simulink subsystem "PvtSubSys_PLAN_ALC"  (R2020b)
settings: Solver=VariableStepAuto  StartTime=0.0  StopTime=10.0  RelTol=1e-3
undefined symbols (not defined in the file or in its folder): P_Global_WheelBase_m, P_Global_WheelTrack_m, P_PLAN_ALC_DPCConfirmTimeHMI, P_PLAN_ALC_DPCExtraMultiFrameConfirmCntDrv, P_PLAN_ALC_DPCExtraMultiFrameConfirmCntNoh, P_PLAN_ALC_DPCExtraMultiFrameConfirmCntOverTk, P_PLAN_ALC_DPCthresholdLcDrvLv1, P_PLAN_ALC_DPCthresholdLcDrvLv2, P_PLAN_ALC_DPCthresholdLcDrvLv3, P_PLAN_ALC_DynamicDPCthreshold, P_PLAN_ALC_FWheelPreTime, P_PLAN_ALC_LcCancelDPCThreshold, P_PLAN_ALC_LcCancelLaneChangeReqDspTimeCnt, P_PLAN_ALC_LcCancelRoadWidthOffset, P_PLAN_ALC_LcCancelRoadWidthOffsetForDPC, P_PLAN_ALC_LcCurvatureInhibitionValueBrkPoints, P_PLAN_ALC_LcCurvatureInhibitionValueTable, P_PLAN_ALC_LcDelayCntSetNoh, P_PLAN_ALC_LcDelayCntSetOverTk, P_PLAN_ALC_LCDeltaTmeGap, P_PLAN_ALC_LcDrv_DyDiffThreshold, P_PLAN_ALC_LcDrvHMILineValidFtime, P_PLAN_ALC_LcEnterLane_factor, P_PLAN_ALC_LcFinishDyDiffBrkPoint, P_PLAN_ALC_LcFinishDyDiffRwFactorForAP, P_PLAN_ALC_LcFinishDyDiffRwFactorForHMI, P_PLAN_ALC_LcFinishDyDiffTableValue, P_PLAN_ALC_LciDrvExistDefaultDisp, P_PLAN_ALC_LciOverTkDeltaSpdLv1, P_PLAN_ALC_LciOverTkDeltaSpdLv2, P_PLAN_ALC_LciOverTkDeltaSpdLv3, P_PLAN_ALC_LcOverTkDPCthreshold, P_PLAN_ALC_LcOverTkRearVehTTClimit, P_PLAN_ALC_NOHLcSwt, P_PLAN_ALC_NOHTurnSts, P_PLAN_ALC_OverTkCutOutDyRWFactor, P_PLAN_ALC_OveTkrSupDist, P_PLAN_ALC_PreCurvatureFactor, P_PLAN_ALC_PreCurvaturePreTime, P_PLAN_ALC_TurnLmpType, P_PLAN_ALC_vMinPreLC_Drv, P_PLAN_ALC_vMinPreLC_Noh, P_PLAN_ALC_vMinPreLC_OverTk, P_PLAN_LcCancelTestEnable, PLAN_ALC_DangerObjIndex, PLAN_ALC_LcCancelReason, PLAN_ALC_LcDecsLe, PLAN_ALC_LcDecsRi, PLAN_ALC_LcFeReason, PLAN_ALC_LcReason, PLAN_ALC_sts, PLAN_ALC_stsReason, PLAN_ALC_TurnLightReq
libraries: simulink x198, TrueDurationTime x21, RisingEdgeTimer x2, JumpDetectionUint x1
(part 2 of 4)

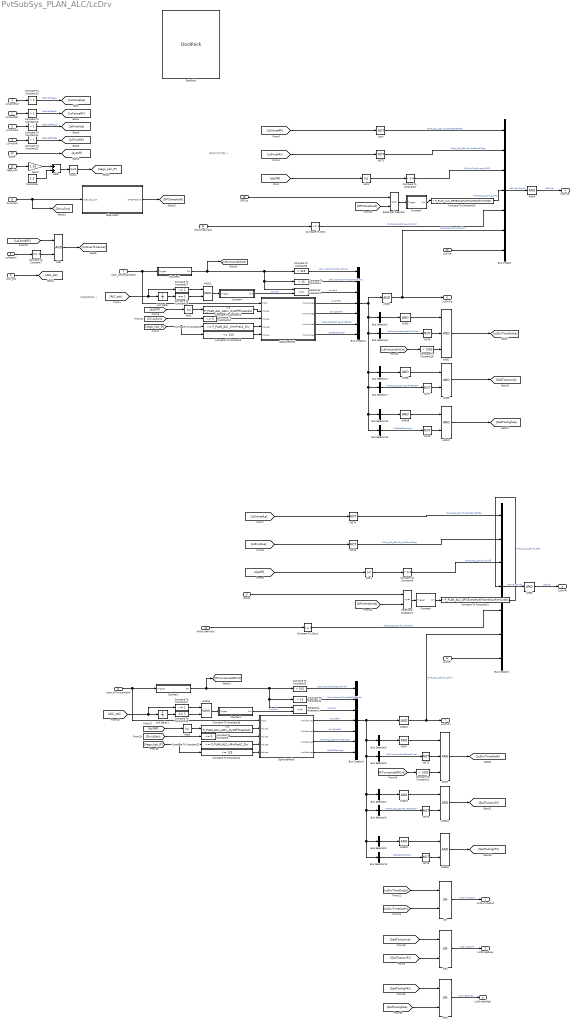
== system PvtSubSys_PLAN_ALC/LcDrv ==
  note: 换道可行性判断->
  note: 换道意图判断->
  LcCancelLe : Inport
  LcCancelRi : Inport  Port=2
  LcFinishLe : Inport  Port=3
  LcFinishRi : Inport  Port=4
  LcReason : Inport  Port=5
  ALC_sts : Inport  Port=6
  User_LeTurnLampON : Inport  Port=7
  User_RiTurnLampON : Inport  Port=8
  DrvLcSwt : Inport  Port=9
  dyDiff : Inport  Port=10
  HWALineLValid : Inport  Port=11
  HWALineRValid : Inport  Port=12
  LcAvLe : Inport  Port=13
  LcAvRi : Inport  Port=14
  Vego_kph : Inport  Port=15
  DPCLe : Inport  Port=16
  DPCRi : Inport  Port=17
  AND{,5,12,15,17} (5 alike) : Logic  AllPortsSameDT=off  OutDataTypeStr=boolean
  AND1 : Logic  Inputs=3  AllPortsSameDT=off  OutDataTypeStr=boolean
  AND{3,7..10,13,16,18} (8 alike) : Logic  Inputs=1  AllPortsSameDT=off  OutDataTypeStr=boolean
  AND11 : Logic  Operator=NAND  AllPortsSameDT=off  OutDataTypeStr=boolean
  AND14 : Logic  Operator=NAND  AllPortsSameDT=off  OutDataTypeStr=boolean
  AND2 : Logic  Inputs=3  AllPortsSameDT=off  OutDataTypeStr=boolean
  AND4 : Logic  Inputs=1  IconShape=distinctive  AllPortsSameDT=off  OutDataTypeStr=boolean
  AND6 : Logic  Inputs=1  IconShape=distinctive  AllPortsSameDT=off  OutDataTypeStr=boolean
  Abs{1..2,4..5} (4 alike) : Abs
  Add2 : Sum
  Bus Creator{,1..3} (4 alike) : BusCreator  Inputs=7
  Bus Selector1 : BusSelector  OutputSignals=LeTurnLampOnTimeNotTooShort,LciValid,DrvLcSwtON,PLAN_ALC_LcDrvLe_IPVehSpd,SpdNotTooHigh  OutputAsBus=on
  Bus Selector10 : BusSelector  OutputSignals=SpdNotTooHigh
  Bus Selector{2,4,9,11} (4 alike) : BusSelector  OutputSignals=LeTurnLampOnNotOverTime,LeTurnLampOnTimeNotTooShort,LciValid,DrvLcSwtON  OutputAsBus=on
  Bus Selector12 : BusSelector  OutputSignals=SpdNotTooHigh
  Bus Selector3 : BusSelector  OutputSignals=LeTurnLampOnTimeNotTooShort,LciValid,DrvLcSwtON,PLAN_ALC_LcDrvRi_IPVehSpd,SpdNotTooHigh  OutputAsBus=on
  Bus Selector5 : BusSelector  OutputSignals=PLAN_ALC_LcDrvRi_IPVehSpd
  Bus Selector6 : BusSelector  OutputSignals=LeTurnLampOnNotOverTime
  Bus Selector7 : BusSelector  OutputSignals=PLAN_ALC_LcDrvLe_IPVehSpd
  Bus Selector8 : BusSelector  OutputSignals=LeTurnLampOnNotOverTime
  Compare To Constant1 : simulink/Logic and Bit Operations/Compare To Constant  relop=<=  const=P_PLAN_ALC_LcDrv_DyDiffThreshold  OutDataTypeStr=boolean
  Compare To Constant10 : simulink/Logic and Bit Operations/Compare To Constant  relop=~=  const=0  OutDataTypeStr=boolean
  Compare To Constant11 : simulink/Logic and Bit Operations/Compare To Constant  relop=<  const=1000  OutDataTypeStr=boolean
  Compare To Constant12 : simulink/Logic and Bit Operations/Compare To Constant  relop=<=  const=125  OutDataTypeStr=boolean
  Compare To Constant{13..15,22} (4 alike) : simulink/Logic and Bit Operations/Compare To Constant  relop=>  const=1  OutDataTypeStr=boolean
  Compare To Constant16 : simulink/Logic and Bit Operations/Compare To Constant  relop=<  const=1000  OutDataTypeStr=boolean
  Compare To Constant17 : simulink/Logic and Bit Operations/Compare To Constant  relop=~=  const=1  OutDataTypeStr=boolean
  Compare To Constant18 : simulink/Logic and Bit Operations/Compare To Constant  relop=<=  const=P_PLAN_ALC_LcDrv_DyDiffThreshold  OutDataTypeStr=boolean
  Compare To Constant19 : simulink/Logic and Bit Operations/Compare To Constant  relop===  const=1  OutDataTypeStr=boolean
  Compare To Constant2 : simulink/Logic and Bit Operations/Compare To Constant  relop=>=  const=P_PLAN_ALC_vMinPreLC_Drv  OutDataTypeStr=boolean
  Compare To Constant20 : simulink/Logic and Bit Operations/Compare To Constant  relop=>  const=P_PLAN_ALC_DPCExtraMultiFrameConfirmCntDrv  OutDataTypeStr=boolean
  Compare To Constant21 : simulink/Logic and Bit Operations/Compare To Constant  relop=>  const=P_PLAN_ALC_DPCExtraMultiFrameConfirmCntDrv  OutDataTypeStr=boolean
  Compare To Constant23 : simulink/Logic and Bit Operations/Compare To Constant  relop=>=  const=P_PLAN_ALC_vMinPreLC_Drv  OutDataTypeStr=boolean
  Compare To Constant24 : simulink/Logic and Bit Operations/Compare To Constant  relop=>  const=15  OutDataTypeStr=boolean
  Compare To Constant25 : simulink/Logic and Bit Operations/Compare To Constant  relop=<  const=515  OutDataTypeStr=boolean
  Compare To Constant27 : simulink/Logic and Bit Operations/Compare To Constant  relop=~=  const=1  OutDataTypeStr=boolean
  Compare To Constant28 : simulink/Logic and Bit Operations/Compare To Constant  relop===  const=1  OutDataTypeStr=boolean
  Compare To Constant3 : simulink/Logic and Bit Operations/Compare To Constant  relop=<=  const=125  OutDataTypeStr=boolean
  Compare To Constant4 : simulink/Logic and Bit Operations/Compare To Constant  relop=>  const=15  OutDataTypeStr=boolean
  Compare To Constant5 : simulink/Logic and Bit Operations/Compare To Constant  relop=<  const=0.4  OutDataTypeStr=boolean
  Compare To Constant6 : simulink/Logic and Bit Operations/Compare To Constant  relop=<  const=0.4  OutDataTypeStr=boolean
  Compare To Constant7 : simulink/Logic and Bit Operations/Compare To Constant  relop===  const=4  OutDataTypeStr=boolean
  Compare To Constant8 : simulink/Logic and Bit Operations/Compare To Constant  relop=<  const=515  OutDataTypeStr=boolean
  Compare To Constant9 : simulink/Logic and Bit Operations/Compare To Constant  relop=~=  const=0  OutDataTypeStr=boolean
  Compare To Zero : simulink/Logic and Bit Operations/Compare To Zero  relop=~=  OutDataTypeStr=boolean
  Compare To Zero1 : simulink/Logic and Bit Operations/Compare To Zero  relop=~=  OutDataTypeStr=boolean
  Constant6 : Constant  Value=1.3  OutDataTypeStr=single
  Counter1 : Subsystem
  Counter2 : Subsystem
  Counter3 : Subsystem
  Counter4 : Subsystem
  Counter5 : Subsystem
  Counter6 : Subsystem
  DocBlock : simulink/Model-Wide Utilities/DocBlock  DocumentType=Text
      content=|
      | 模块说明：
      | 该模块用于计算是否触发拨杆换道，换道条件如下：
      |
      | 当如下条件全部满足左换道可行
      | 1.手动换道开关开启；
      | 2.车身中心距离车道中心线0.4m以内；
      | 3.仪表车速大于等于40kmh；
      | 4.左侧车道安全，换道过程中无碰撞风险；
      | 5.左侧车道控制线有效；
      | 6.3s内未发生右换道取消；
      | 7.3s内未发生右换道完成；
      | 8.左侧转向灯开关开启时（上升沿）开始计时，关闭左转向灯时或车辆中心距离控制线>0.8m或状态跳转到非Cruise（上升沿）时停止计时，计时满0.3s但不超过10s；
      |
      | 当如下条件全部满足则满足右换道可行
      | 1.手动换道开关开启；
      | 2.车身中心距离本车道中心线0.4m以内；
      | 3.仪表车速大于等于40kmh；
      | 4.左侧车道安全，换道过程中无碰撞风险；
      | 5.左侧车道控制线有效；
      | 6.3s内未发生左换道取消；
      | 7.3s内未发生左换道完成；
      | 8.右侧转向灯开关开启时（上升沿）开始计时，关闭右转向灯时或车辆中心距离控制线>0.8m或状态跳转到非Cruise（上升沿）时停止计时，计时满0.3s但不超过10s；
  Gain2 : Gain  Gain=1.03
  NOT{,1..9} (10 alike) : Logic  Operator=NOT  IconShape=distinctive  AllPortsSameDT=off  OutDataTypeStr=boolean
  OR : Logic  Operator=OR  AllPortsSameDT=off  OutDataTypeStr=boolean
  OR1 : Logic  Operator=OR  AllPortsSameDT=off  OutDataTypeStr=boolean
  OR2 : Logic  Operator=OR  AllPortsSameDT=off  OutDataTypeStr=boolean
  Relational Operator{,1..3} (4 alike) : RelationalOperator  Operator=<=  OutDataTypeStr=boolean  RndMeth=Simplest
  Round : Rounding  Operator=round
  SigValueHold1 : Stateflow chart  TreatAsAtomicUnit=on
  SigValueHold3 : Stateflow chart  TreatAsAtomicUnit=on
  Subsystem : Subsystem
  Unit Delay : UnitDelay  SampleTime=-1  HasFrameUpgradeWarning=on
  Unit Delay1 : UnitDelay  SampleTime=-1  HasFrameUpgradeWarning=on
  LciDrvTimeOut : Outport
  LciDrvSpdLow : Outport  Port=2
  LciDrvSpdHigh : Outport  Port=3
  LcDrvLe : Outport  Port=4
  LcDrvRi : Outport  Port=5
  LciDrvLe : Outport  Port=6
  LciDrvRi : Outport  Port=7
  wires:
  LcAvRi/1 -> Bus Creator1/7
  LcAvLe/1 -> Bus Creator/7
  OR2/1 -> LciDrvSpdHigh/1  "LciDrvSpdHigh"
  [SpdToohighLe] -> OR2/2
  [SpdToohighRi] -> OR2/1
  AND18/1 -> AND17/1
  NOT9/1 -> AND17/2
  Bus Selector11/1 -> AND18/1
  Bus Selector12/1 -> NOT9/1  "<SpdNotTooHigh>"
  AND17/1 -> [SpdToohighLe]
  Bus Creator2/1 -> AND3/1, Bus Selector1/1, Bus Selector8/1, Bus Selector2/1, Bus Selector7/1, Bus Selector11/1, Bus Selector12/1
  Bus Creator3/1 -> Bus Selector3/1, Bus Selector6/1, Bus Selector4/1, Bus Selector5/1, Bus Selector10/1, Bus Selector9/1, AND10/1
  AND15/1 -> [SpdToohighRi]
  Bus Selector10/1 -> NOT8/1  "<SpdNotTooHigh>"
  Bus Selector9/1 -> AND16/1
  NOT8/1 -> AND15/2
  AND16/1 -> AND15/1
  AND/1 -> [LcOverTkCancel]
  Compare To Constant7/1 -> AND/2
  [LcCancelRi] -> AND/1
  LcReason/1 -> Compare To Constant7/1
  Bus Creator1/1 -> AND6/1  "LcDrvRi_Conds"
  AND6/1 -> LcDrvRi/1  "LcDrvRi"
  AND4/1 -> LcDrvLe/1  "LcDrvLe"
  OR/1 -> LciDrvTimeOut/1  "LciDrvTimeOut"
  [LciDrvTimeOutRi] -> OR/2
  [LciDrvTimeOutLe] -> OR/1
  Bus Creator/1 -> AND4/1  "LcDrvLe_Conds"
  [LcFinishLe] -> NOT5/1
  [LcCancelLe] -> NOT4/1
  [LcFinishRi] -> NOT1/1
  NOT/1 -> Bus Creator/1  "PLAN_ALC_LcDrvLe_NoLcCancelFlag"
  LcFinishLe/1 -> Compare To Constant14/1
  LcFinishRi/1 -> Compare To Constant22/1
  LcCancelRi/1 -> Compare To Constant15/1
  Compare To Constant5/1 -> Bus Creator1/3  "PLAN_ALC_LcDrvRi_dyDiff"
  Abs4/1 -> Compare To Constant5/1
  [dyDiff] -> Abs4/1
  NOT5/1 -> Bus Creator1/2  "PLAN_ALC_LcDrvRi_NoLcFinishFlag"
  NOT4/1 -> Bus Creator1/1  "PLAN_ALC_LcDrvRi_NoLcCancelFlag"
  NOT1/1 -> Bus Creator/2  "PLAN_ALC_LcDrvLe_NoLcFinishFlag"
  [LcCancelRi] -> NOT/1
  [dyDiff] -> Abs1/1
  dyDiff/1 -> [dyDiff]
  LcCancelLe/1 -> Compare To Constant13/1
  HWALineRValid/1 -> Compare To Zero1/1
  Abs1/1 -> Compare To Constant6/1
  Compare To Constant6/1 -> Bus Creator/3  "PLAN_ALC_LcDrvLe_dyDiff"
  Compare To Constant20/1 -> Bus Creator/4  "PLAN_ALC_LcDrvLe_DPC"
  HWALineLValid/1 -> Compare To Zero/1
  [DPCthreshold] -> Relational Operator1/2
  Compare To Zero1/1 -> Bus Creator1/5  "PLAN_ALC_LcDrvRi_LineValid"
  Relational Operator1/1 -> Counter6/1(Trigger)
  DPCLe/1 -> Relational Operator/1
  DPCRi/1 -> Relational Operator1/1
  [DPCthreshold] -> Relational Operator/2
  Compare To Zero/1 -> Bus Creator/5  "PLAN_ALC_LcDrvLe_LineValid"
  [SpdTooLowLe] -> OR1/1
  [SpdTooLowRi] -> OR1/2
  OR1/1 -> LciDrvSpdLow/1  "LciDrvSpdLow"
  Compare To Constant13/1 -> [LcCancelLe]  "LcFinishFlagLe"
  Compare To Constant15/1 -> [LcCancelRi]  "LcFinishFlagRi"
  Compare To Constant14/1 -> [LcFinishLe]  "LcCancelFlagLe"
  Compare To Constant22/1 -> [LcFinishRi]  "LcCancelFlagRi"
  Constant6/1 -> Add2/2
  Gain2/1 -> Add2/1
  Add2/1 -> Round/1
  Vego_kph/1 -> Gain2/1
  DrvLcSwt/1 -> [DrvLcSwt], Subsystem/1(User_ALC_Swt)
  Round/1 -> [Vego_kph_IP]
  AND13/1 -> AND12/1
  NOT3/1 -> AND12/2
  Bus Selector4/1 -> AND13/1
  Bus Selector5/1 -> NOT3/1  "<PLAN_ALC_LcDrvRi_IPVehSpd>"
  SigValueHold3/3(HoldValue3) -> Bus Creator3/6  "PLAN_ALC_LcDrvRi_IPVehSpd"
  Compare To Constant23/1 -> SigValueHold3/4(Value3)
  [DrvLcSwt] -> Compare To Constant9/1
  Compare To Constant18/1 -> SigValueHold3/2(Value1)
  SigValueHold3/2(HoldValue2) -> Bus Creator3/5  "DrvLcSwtON"
  Compare To Constant24/1 -> Bus Creator3/2  "LeTurnLampOnTimeNotTooShort"
  Compare To Constant25/1 -> Bus Creator3/1  "LeTurnLampOnNotOverTime"
  [dyDiff] -> Abs5/1
  Counter1/1(Cnt) -> [RiTurnLampONCnt], Compare To Constant24/1, Relational Operator2/1, Compare To Constant25/1
  AND12/1 -> [SpdTooLowRi]
  User_RiTurnLampON/1 -> SigValueHold3/1(Hold), Counter1/1(Trigger)
  AND10/1 -> LciDrvRi/1, Bus Creator1/6  "PLAN_ALC_LcDrvRi_LciDrv"
  SigValueHold3/1(HoldValue1) -> Bus Creator3/4  "DyDiffOK"
  Abs5/1 -> Compare To Constant18/1
  Compare To Constant9/1 -> SigValueHold3/3(Value2)
  ALC_sts/1 -> [ALC_sts]
  Relational Operator2/1 -> Bus Creator3/3  "LciValid"
  Bus Selector6/1 -> NOT2/1  "<LeTurnLampOnNotOverTime>"
  Bus Selector3/1 -> AND7/1
  NOT2/1 -> AND1/2
  AND7/1 -> AND1/1
  AND1/1 -> [LciDrvTimeOutRi]
  AND2/1 -> [LciDrvTimeOutLe]
  AND9/1 -> AND2/1
  NOT6/1 -> AND2/2
  Bus Selector1/1 -> AND9/1
  Bus Selector8/1 -> NOT6/1  "<LeTurnLampOnNotOverTime>"
  Relational Operator3/1 -> Bus Creator2/3  "LciValid"
  Compare To Constant10/1 -> SigValueHold1/3(Value2)
  Abs2/1 -> Compare To Constant1/1
  SigValueHold1/1(HoldValue1) -> Bus Creator2/4  "DyDiffOK"
  AND3/1 -> LciDrvLe/1, Bus Creator/6  "PLAN_ALC_LcDrvLe_LciDrv"
  User_LeTurnLampON/1 -> Counter2/1(Trigger), SigValueHold1/1(Hold)
  AND5/1 -> [SpdTooLowLe]
  Counter2/1(Cnt) -> Compare To Constant4/1, Relational Operator3/1, Compare To Constant8/1, [LeTurnLampONCnt]
  [Vego_kph_IP] -> Compare To Constant3/1, Compare To Constant2/1
  [dyDiff] -> Abs2/1
  Compare To Constant8/1 -> Bus Creator2/1  "LeTurnLampOnNotOverTime"
  Compare To Constant4/1 -> Bus Creator2/2  "LeTurnLampOnTimeNotTooShort"
  SigValueHold1/2(HoldValue2) -> Bus Creator2/5  "DrvLcSwtON"
  Compare To Constant1/1 -> SigValueHold1/2(Value1)
  [DrvLcSwt] -> Compare To Constant10/1
  Compare To Constant2/1 -> SigValueHold1/4(Value3)
  SigValueHold1/3(HoldValue3) -> Bus Creator2/6  "PLAN_ALC_LcDrvLe_IPVehSpd"
  Bus Selector7/1 -> NOT7/1  "<PLAN_ALC_LcDrvLe_IPVehSpd>"
  Bus Selector2/1 -> AND8/1
  NOT7/1 -> AND5/2
  AND8/1 -> AND5/1
  [RiTurnLampONCnt] -> Compare To Constant11/1
  Compare To Constant11/1 -> AND1/3
  [LeTurnLampONCnt] -> Compare To Constant16/1
  Compare To Constant16/1 -> AND2/3
  Compare To Constant27/1 -> AND11/1
  [ALC_sts] -> Compare To Constant27/1, Unit Delay/1
  Compare To Constant28/1 -> AND11/2
  Unit Delay/1 -> Compare To Constant28/1
  AND11/1 -> Counter4/1(Trigger)
  AND14/1 -> Counter3/1(Trigger)
  Unit Delay1/1 -> Compare To Constant19/1
  Compare To Constant19/1 -> AND14/2
  [ALC_sts] -> Compare To Constant17/1, Unit Delay1/1
  Compare To Constant17/1 -> AND14/1
  Counter3/1(Cnt) -> Relational Operator2/2  "LciValid"
  Counter4/1(Cnt) -> Relational Operator3/2  "LciValid"
  Subsystem/1(DPCthreshold) -> [DPCthreshold]
  Compare To Constant3/1 -> SigValueHold1/5(Value4)
  SigValueHold1/4(HoldValue4) -> Bus Creator2/7  "SpdNotTooHigh"
  Compare To Constant12/1 -> SigValueHold3/5(Value4)
  [Vego_kph_IP] -> Compare To Constant12/1, Compare To Constant23/1
  SigValueHold3/4(HoldValue4) -> Bus Creator3/7  "SpdNotTooHigh"
  Relational Operator/1 -> Counter5/1(Trigger)
  Counter5/1(Cnt) -> Compare To Constant20/1
  Compare To Constant21/1 -> Bus Creator1/4  "PLAN_ALC_LcDrvRi_DPC"
  Counter6/1(Cnt) -> Compare To Constant21/1

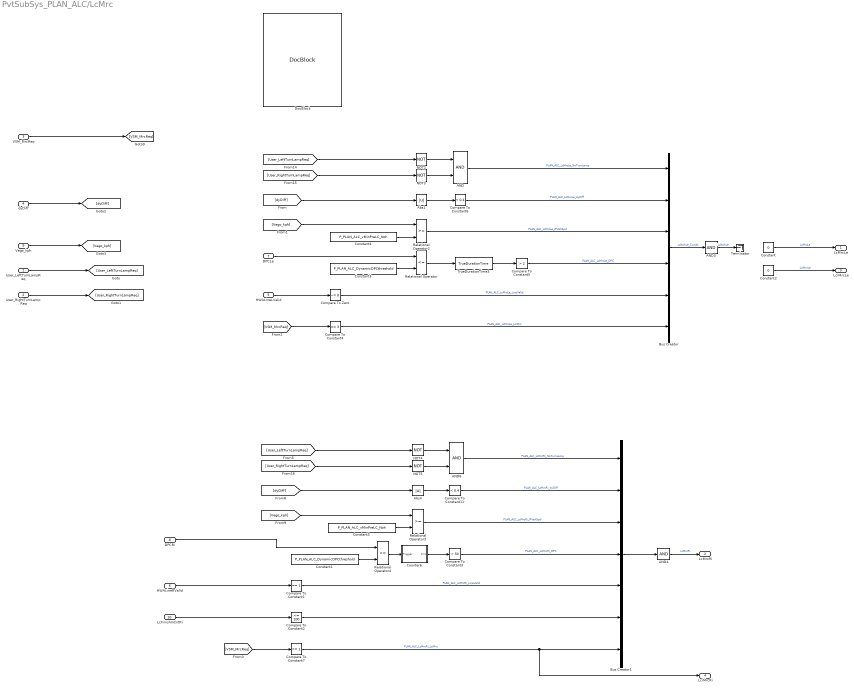
== system PvtSubSys_PLAN_ALC/LcMrc ==
  User_LeftTurnLampReq : Inport
  User_RightTurnLampReq : Inport  Port=2
  VSM_MrcReq : Inport  Port=3
  dyDiff : Inport  Port=4
  HWALineLValid : Inport  Port=5
  HWALineRValid : Inport  Port=6
  DPCLe : Inport  Port=7
  DPCRi : Inport  Port=8
  Vego_kph : Inport  Port=9
  LcFinishInCntRi : Inport  Port=10
  AND : Logic  AllPortsSameDT=off  OutDataTypeStr=boolean
  AND3 : Logic  Inputs=1  AllPortsSameDT=off  OutDataTypeStr=boolean
  AND4 : Logic  Inputs=1  AllPortsSameDT=off  OutDataTypeStr=boolean
  AND6 : Logic  AllPortsSameDT=off  OutDataTypeStr=boolean
  Abs1 : Abs
  Abs4 : Abs
  Bus Creator : BusCreator  Inputs=6
  Bus Creator1 : BusCreator  Inputs=7
  Compare To Constant1 : simulink/Logic and Bit Operations/Compare To Constant  relop===  const=1  OutDataTypeStr=boolean
  Compare To Constant11 : simulink/Logic and Bit Operations/Compare To Constant  relop=<  const=0.4  OutDataTypeStr=boolean
  Compare To Constant2 : simulink/Logic and Bit Operations/Compare To Constant  relop=<=  const=100  OutDataTypeStr=boolean
  Compare To Constant3 : simulink/Logic and Bit Operations/Compare To Constant  relop=>  const=50  OutDataTypeStr=boolean
  Compare To Constant4 : simulink/Logic and Bit Operations/Compare To Constant  relop===  const=3  OutDataTypeStr=boolean
  Compare To Constant5 : simulink/Logic and Bit Operations/Compare To Constant  relop=>  const=2  OutDataTypeStr=boolean
  Compare To Constant6 : simulink/Logic and Bit Operations/Compare To Constant  relop=<  const=0.4  OutDataTypeStr=boolean
  Compare To Constant7 : simulink/Logic and Bit Operations/Compare To Constant  relop===  const=1  OutDataTypeStr=boolean
  Compare To Zero : simulink/Logic and Bit Operations/Compare To Zero  relop=~=  OutDataTypeStr=boolean
  Constant : Constant  Value=0  OutDataTypeStr=boolean
  Constant1 : Constant  Value=P_PLAN_ALC_DynamicDPCthreshold
  Constant2 : Constant  Value=0  OutDataTypeStr=boolean
  Constant3 : Constant  Value=P_PLAN_ALC_DynamicDPCthreshold
  Constant4 : Constant  Value=P_PLAN_ALC_vMinPreLC_Noh
  Constant5 : Constant  Value=P_PLAN_ALC_vMinPreLC_Noh
  Counter6 : Subsystem
  DocBlock : simulink/Model-Wide Utilities/DocBlock  DocumentType=Text
      content=|
      | 模块说明：
      | 该模块用于计算是否触发NOH换道，换道条件如下：
      |
      | 当如下条件全部满足进入左换道状态
      | 1.车身中心距离车道中心线0.4m以内；
      | 2.仪表车速大于等于40kmh；
      | 3.左侧车道安全，换道过程中无碰撞风险；
      | 4.左侧车道控制线有效持续5帧；
      | 5.NOH请求左换道>1.5s；
      | 6.驾驶员未开启转向灯；
      | 7.3s内未发生左换道成功；
      |
      | 当如下条件全部满足进入右换道状态
      | 1.车身中心距离车道中心线0.4m以内；
      | 2.仪表车速大于等于40kmh；
      | 3.右侧车道安全，换道过程中无碰撞风险；
      | 4.右侧车道控制线有效持续5帧；
      | 5.NOH请求左换道>1.5s；
      | 6.驾驶员未开启转向灯；
      | 7.3s内未发生右换道成功；
  NOT{2..5} (4 alike) : Logic  Operator=NOT  IconShape=distinctive  AllPortsSameDT=off  OutDataTypeStr=boolean
  Relational Operator : RelationalOperator  Operator=<=  OutDataTypeStr=boolean  RndMeth=Simplest
  Relational Operator2 : RelationalOperator  OutDataTypeStr=boolean  RndMeth=Simplest
  Relational Operator3 : RelationalOperator  OutDataTypeStr=boolean  RndMeth=Simplest
  Relational Operator4 : RelationalOperator  Operator=<=  OutDataTypeStr=boolean  RndMeth=Simplest
  Terminator : Terminator
  TrueDurationTime3 : TrueDurationTime/TrueDurationTime  TCycle=0.02
  LcMrcLe : Outport
  LcMrcRi : Outport  Port=2
  LciMrcLe : Outport  Port=3
  LciMrcRi : Outport  Port=4
  wires:
  Constant2/1 -> LciMrcLe/1  "LciMrcLe"
  DPCRi/1 -> Relational Operator4/1
  Constant1/1 -> Relational Operator4/2
  Constant/1 -> LcMrcLe/1  "LcMrcLe"
  AND3/1 -> Terminator/1  "LcNohLe"
  [User_LeftTurnLampReq] -> NOT4/1
  [User_RightTurnLampReq] -> NOT5/1
  NOT4/1 -> AND6/1
  NOT5/1 -> AND6/2
  NOT3/1 -> AND/2
  NOT2/1 -> AND/1
  [User_RightTurnLampReq] -> NOT3/1
  [User_LeftTurnLampReq] -> NOT2/1
  AND6/1 -> Bus Creator1/1  "PLAN_ALC_LcMrcRi_NoTurnLamp"
  AND/1 -> Bus Creator/1  "PLAN_ALC_LcMrcLe_NoTurnLamp"
  Compare To Constant1/1 -> Bus Creator1/5  "PLAN_ALC_LcMrcRi_LineValid"
  dyDiff/1 -> [dyDiff]
  TrueDurationTime3/1 -> Compare To Constant5/1
  Relational Operator3/1 -> Bus Creator1/3  "PLAN_ALC_LcMrcRi_IPVehSpd"
  [Vego_kph] -> Relational Operator3/1
  Abs1/1 -> Compare To Constant6/1
  Relational Operator/1 -> TrueDurationTime3/1
  HWALineLValid/1 -> Compare To Zero/1
  Constant4/1 -> Relational Operator2/2
  [Vego_kph] -> Relational Operator2/1
  DPCLe/1 -> Relational Operator/1
  User_LeftTurnLampReq/1 -> [User_LeftTurnLampReq]
  Constant3/1 -> Relational Operator/2
  Bus Creator/1 -> AND3/1  "LcNohLe_Conds"
  [dyDiff] -> Abs1/1
  Compare To Constant5/1 -> Bus Creator/4  "PLAN_ALC_LcMrcLe_DPC"
  Relational Operator2/1 -> Bus Creator/3  "PLAN_ALC_LcMrcLe_IPVehSpd"
  Relational Operator4/1 -> Counter6/1(Trigger)
  Vego_kph/1 -> [Vego_kph]
  Abs4/1 -> Compare To Constant11/1
  [VSM_MrcReq] -> Compare To Constant4/1
  User_RightTurnLampReq/1 -> [User_RightTurnLampReq]
  Constant5/1 -> Relational Operator3/2
  Compare To Constant11/1 -> Bus Creator1/2  "PLAN_ALC_LcMrcRi_dyDiff"
  [VSM_MrcReq] -> Compare To Constant7/1
  VSM_MrcReq/1 -> [VSM_MrcReq]
  Compare To Constant4/1 -> Bus Creator/6  "PLAN_ALC_LcMrcLe_LciMrc"
  [dyDiff] -> Abs4/1
  AND4/1 -> LcMrcRi/1  "LcMrcRi"
  HWALineRValid/1 -> Compare To Constant1/1
  Compare To Constant7/1 -> Bus Creator1/7, LciMrcRi/1  "PLAN_ALC_LcMrcRi_LciMrc"
  Compare To Constant6/1 -> Bus Creator/2  "PLAN_ALC_LcMrcLe_dyDiff"
  Compare To Zero/1 -> Bus Creator/5  "PLAN_ALC_LcMrcLe_LineValid"
  Bus Creator1/1 -> AND4/1
  LcFinishInCntRi/1 -> Compare To Constant2/1
  Compare To Constant2/1 -> Bus Creator1/6
  Compare To Constant3/1 -> Bus Creator1/4  "PLAN_ALC_LcMrcRi_DPC"
  Counter6/1(Cnt) -> Compare To Constant3/1

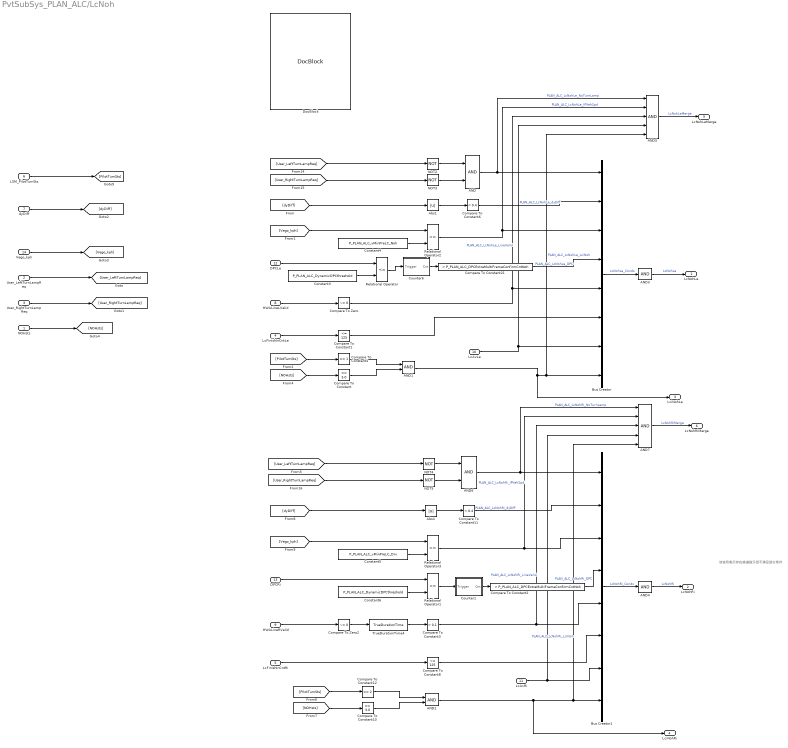
== system PvtSubSys_PLAN_ALC/LcNoh ==
  note: 该信号表示存在换道指示但不满足部分条件
  NOHsts : Inport
  User_LeftTurnLampReq : Inport  Port=2
  User_RightTurnLampReq : Inport  Port=3
  LcFinishInCntLe : Inport  Port=4
  LcFinishInCntRi : Inport  Port=5
  LSM_PilotTurnSts : Inport  Port=6
  dyDiff : Inport  Port=7
  HWALineLValid : Inport  Port=8
  HWALineRValid : Inport  Port=9
  LcAvLe : Inport  Port=10
  LcAvRi : Inport  Port=11
  DPCLe : Inport  Port=12
  DPCRi : Inport  Port=13
  Vego_kph : Inport  Port=14
  AND{,1..2,6} (4 alike) : Logic  AllPortsSameDT=off  OutDataTypeStr=boolean
  AND3 : Logic  Inputs=1  AllPortsSameDT=off  OutDataTypeStr=boolean
  AND4 : Logic  Inputs=1  AllPortsSameDT=off  OutDataTypeStr=boolean
  AND5 : Logic  Inputs=5  AllPortsSameDT=off  OutDataTypeStr=boolean
  AND7 : Logic  Inputs=5  AllPortsSameDT=off  OutDataTypeStr=boolean
  Abs1 : Abs
  Abs4 : Abs
  Bus Creator : BusCreator  Inputs=8
  Bus Creator1 : BusCreator  Inputs=8
  Compare To Constant : simulink/Logic and Bit Operations/Compare To Constant  relop===  const=3.0  OutDataTypeStr=boolean
  Compare To Constant1 : simulink/Logic and Bit Operations/Compare To Constant  relop=<=  const=125  OutDataTypeStr=boolean
  Compare To Constant10 : simulink/Logic and Bit Operations/Compare To Constant  relop===  const=3.0  OutDataTypeStr=boolean
  Compare To Constant11 : simulink/Logic and Bit Operations/Compare To Constant  relop=<  const=0.4  OutDataTypeStr=boolean
  Compare To Constant12 : simulink/Logic and Bit Operations/Compare To Constant  relop===  const=2  OutDataTypeStr=boolean
  Compare To Constant2 : simulink/Logic and Bit Operations/Compare To Constant  relop=>  const=P_PLAN_ALC_DPCExtraMultiFrameConfirmCntNoh  OutDataTypeStr=boolean
  Compare To Constant21 : simulink/Logic and Bit Operations/Compare To Constant  relop=>  const=P_PLAN_ALC_DPCExtraMultiFrameConfirmCntNoh  OutDataTypeStr=boolean
  Compare To Constant3 : simulink/Logic and Bit Operations/Compare To Constant  relop=>  const=0.1  OutDataTypeStr=boolean
  Compare To Constant4 : simulink/Logic and Bit Operations/Compare To Constant  relop===  const=1  OutDataTypeStr=boolean
  Compare To Constant6 : simulink/Logic and Bit Operations/Compare To Constant  relop=<  const=0.4  OutDataTypeStr=boolean
  Compare To Constant8 : simulink/Logic and Bit Operations/Compare To Constant  relop=<=  const=125  OutDataTypeStr=boolean
  Compare To Zero : simulink/Logic and Bit Operations/Compare To Zero  relop=~=  OutDataTypeStr=boolean
  Compare To Zero2 : simulink/Logic and Bit Operations/Compare To Zero  relop=~=  OutDataTypeStr=boolean
  Constant3 : Constant  Value=P_PLAN_ALC_DynamicDPCthreshold
  Constant4 : Constant  Value=P_PLAN_ALC_vMinPreLC_Noh
  Constant5 : Constant  Value=P_PLAN_ALC_vMinPreLC_Drv
  Constant6 : Constant  Value=P_PLAN_ALC_DynamicDPCthreshold
  Counter1 : Subsystem
  Counter6 : Subsystem
  DocBlock : simulink/Model-Wide Utilities/DocBlock  DocumentType=Text
      content=|
      | 模块说明：
      | 该模块用于计算是否触发NOH换道，换道条件如下：
      |
      | 当如下条件全部满足进入左换道状态
      | 1.车身中心距离车道中心线0.4m以内；
      | 2.仪表车速大于等于40kmh；
      | 3.左侧车道安全，换道过程中无碰撞风险；
      | 4.左侧车道控制线有效持续5帧；
      | 5.NOH请求左换道>1.5s；
      | 6.驾驶员未开启转向灯；
      | 7.3s内未发生左换道成功；
      |
      | 当如下条件全部满足进入右换道状态
      | 1.车身中心距离车道中心线0.4m以内；
      | 2.仪表车速大于等于40kmh；
      | 3.右侧车道安全，换道过程中无碰撞风险；
      | 4.右侧车道控制线有效持续5帧；
      | 5.NOH请求左换道>1.5s；
      | 6.驾驶员未开启转向灯；
      | 7.3s内未发生右换道成功；
  NOT{2..5} (4 alike) : Logic  Operator=NOT  IconShape=distinctive  AllPortsSameDT=off  OutDataTypeStr=boolean
  Relational Operator : RelationalOperator  Operator=<=  OutDataTypeStr=boolean  RndMeth=Simplest
  Relational Operator1 : RelationalOperator  Operator=<=  OutDataTypeStr=boolean  RndMeth=Simplest
  Relational Operator2 : RelationalOperator  OutDataTypeStr=boolean  RndMeth=Simplest
  Relational Operator3 : RelationalOperator  OutDataTypeStr=boolean  RndMeth=Simplest
  TrueDurationTime4 : TrueDurationTime/TrueDurationTime  TCycle=0.02
  LcNohLe : Outport
  LcNohRi : Outport  Port=2
  LciNohLe : Outport  Port=3
  LciNohRi : Outport  Port=4
  LcNohLeMerge : Outport  Port=5
  LcNohRiMerge : Outport  Port=6
  wires:
  AND7/1 -> LcNohRiMerge/1  "LcNohRiMerge"
  AND5/1 -> LcNohLeMerge/1  "LcNohLeMerge"
  LcAvRi/1 -> Bus Creator1/7, AND7/4
  LcAvLe/1 -> Bus Creator/7, AND5/4
  [PilotTurnSts] -> Compare To Constant12/1
  [NOHsts] -> Compare To Constant10/1
  Compare To Constant12/1 -> AND2/1
  Compare To Constant10/1 -> AND2/2
  Compare To Constant/1 -> AND1/2
  Compare To Constant4/1 -> AND1/1
  [NOHsts] -> Compare To Constant/1
  NOHsts/1 -> [NOHsts]
  LcFinishInCntRi/1 -> Compare To Constant8/1
  Compare To Constant8/1 -> Bus Creator1/6
  Compare To Constant1/1 -> Bus Creator/6
  LcFinishInCntLe/1 -> Compare To Constant1/1
  Bus Creator1/1 -> AND4/1  "LcNohRi_Conds"
  Compare To Zero/1 -> Bus Creator/5, AND5/3  "PLAN_ALC_LcNohLe_LineValid"
  Compare To Constant6/1 -> Bus Creator/2  "PLAN_ALC_LcNohLe_dyDiff"
  AND2/1 -> Bus Creator1/8, AND7/5, LciNohRi/1  "PLAN_ALC_LcNohRi_LciNoh"
  TrueDurationTime4/1 -> Compare To Constant3/1
  Compare To Zero2/1 -> TrueDurationTime4/1
  HWALineRValid/1 -> Compare To Zero2/1
  AND4/1 -> LcNohRi/1  "LcNohRi"
  [dyDiff] -> Abs4/1
  AND1/1 -> Bus Creator/8, AND5/5, LciNohLe/1  "PLAN_ALC_LcNohLe_LciNoh"
  LSM_PilotTurnSts/1 -> [PilotTurnSts]
  Compare To Constant11/1 -> Bus Creator1/2  "PLAN_ALC_LcNohRi_dyDiff"
  Constant5/1 -> Relational Operator3/2
  AND3/1 -> LcNohLe/1  "LcNohLe"
  User_RightTurnLampReq/1 -> [User_RightTurnLampReq]
  [PilotTurnSts] -> Compare To Constant4/1
  Abs4/1 -> Compare To Constant11/1
  Vego_kph/1 -> [Vego_kph]
  Compare To Constant2/1 -> Bus Creator1/4  "PLAN_ALC_LcNohRi_DPC"
  Relational Operator2/1 -> Bus Creator/3, AND5/2  "PLAN_ALC_LcNohLe_IPVehSpd"
  Compare To Constant21/1 -> Bus Creator/4  "PLAN_ALC_LcNohLe_DPC"
  [dyDiff] -> Abs1/1
  Bus Creator/1 -> AND3/1  "LcNohLe_Conds"
  Constant3/1 -> Relational Operator/2
  User_LeftTurnLampReq/1 -> [User_LeftTurnLampReq]
  DPCLe/1 -> Relational Operator/1
  [Vego_kph] -> Relational Operator2/1
  Constant4/1 -> Relational Operator2/2
  HWALineLValid/1 -> Compare To Zero/1
  Constant6/1 -> Relational Operator1/2
  Abs1/1 -> Compare To Constant6/1
  [Vego_kph] -> Relational Operator3/1
  DPCRi/1 -> Relational Operator1/1
  Relational Operator3/1 -> Bus Creator1/3, AND7/2  "PLAN_ALC_LcNohRi_IPVehSpd"
  dyDiff/1 -> [dyDiff]
  Compare To Constant3/1 -> Bus Creator1/5, AND7/3  "PLAN_ALC_LcNohRi_LineValid"
  AND/1 -> Bus Creator/1, AND5/1  "PLAN_ALC_LcNohLe_NoTurnLamp"
  AND6/1 -> Bus Creator1/1, AND7/1  "PLAN_ALC_LcNohRi_NoTurnLamp"
  [User_LeftTurnLampReq] -> NOT2/1
  [User_RightTurnLampReq] -> NOT3/1
  NOT2/1 -> AND/1
  NOT3/1 -> AND/2
  NOT5/1 -> AND6/2
  NOT4/1 -> AND6/1
  [User_RightTurnLampReq] -> NOT5/1
  [User_LeftTurnLampReq] -> NOT4/1
  Counter6/1(Cnt) -> Compare To Constant21/1
  Relational Operator/1 -> Counter6/1(Trigger)
  Counter1/1(Cnt) -> Compare To Constant2/1
  Relational Operator1/1 -> Counter1/1(Trigger)

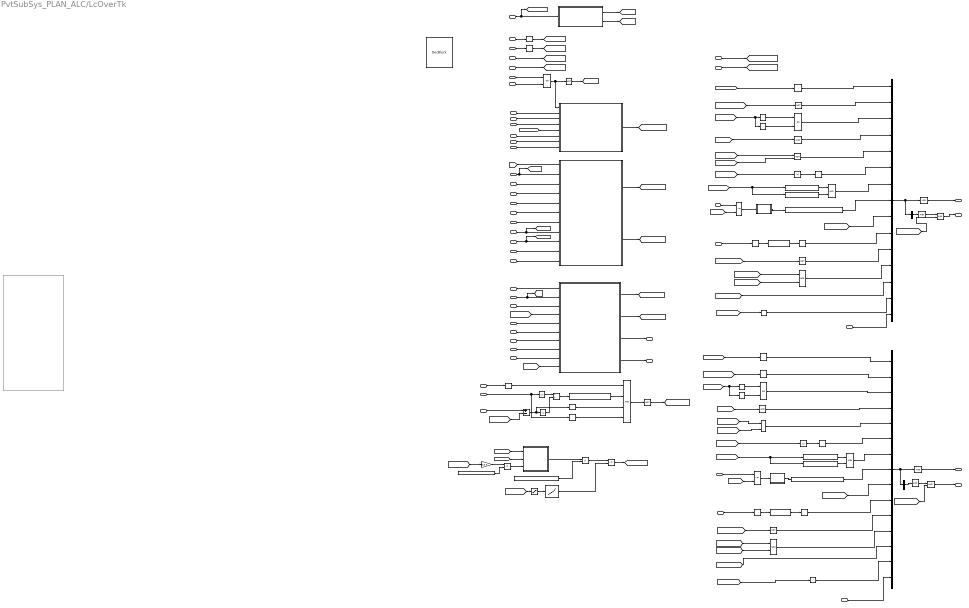
== system PvtSubSys_PLAN_ALC/LcOverTk ==
  User_DrvOverride : Inport
  LCKSts : Inport  Port=2
  SpdSetValue_kph : Inport  Port=3
  P0ID : Inport  Port=4
  P0Vr_ms : Inport  Port=5
  P0Dy : Inport  Port=6
  P0Vy : Inport  Port=7
  P0Dx : Inport  Port=8
  tStartDecel : Inport  Port=9
  NearestObjValid_L : Inport  Port=10
  NearestObjValid_R : Inport  Port=11
  NearestObjSpeed_L : Inport  Port=12
  NearestObjSpeed_R : Inport  Port=13
  Valid : Inport  Port=14
  Dx : Inport  Port=15
  Vx : Inport  Port=16
  DrivingOnTheMostLeftLane_b : Inport  Port=17
  LaneWidth : Inport  Port=18
  HWALineValid : Inport  Port=19
  " HWALineC3" : Inport  Port=20
  HWALineC2 : Inport  Port=21
  HWALineC1 : Inport  Port=22
  HWALineC0 : Inport  Port=23
  HWALineRange : Inport  Port=24
  dyDiff : Inport  Port=25
  HWALineLValid : Inport  Port=26
  HWALineRValid : Inport  Port=27
  LcAvLe : Inport  Port=28
  LcAvRi : Inport  Port=29
  User_ALC_Swt : Inport  Port=30
  LcReason : Inport  Port=31
  LcCancelInCntLe : Inport  Port=32
  LcCancelInCntRi : Inport  Port=33
  User_LeftTurnLampReq : Inport  Port=34
  User_RightTurnLampReq : Inport  Port=35
  DPCLe : Inport  Port=36
  DPCRi : Inport  Port=37
  LcFinishLe : Inport  Port=38
  LcFinishRi : Inport  Port=39
  ALC_sts : Inport  Port=40
  Vego_kph : Inport  Port=41
  LSM_PilotTurnSts : Inport  Port=42
  1-D Lookup Table : Lookup_n-D  NumberOfTableDimensions=1  LookupTableObject=''  BreakpointsForDimension1=P_PLAN_ALC_LcCurvatureInhibitionValueBrkPoints  BreakpointsForDimension1FirstPoint=10  BreakpointsForDimension2FirstPoint=10  BreakpointsForDimension1Spacing=12  BreakpointsForDimension2Spacing=12  IndexSearchMethod=Evenly spaced points  Table=P_PLAN_ALC_LcCurvatureInhibitionValueTable  InterpMethod=Linear Lagrange  ExtrapMethod=Clip  DiagnosticForOutOfRangeInput=Error  UseLastTableValue=on  InternalRulePriority=Speed  RndMeth=Simplest  SaturateOnIntegerOverflow=on  InputSameDT=on
  AND{,2,5,7} (4 alike) : Logic  AllPortsSameDT=off  OutDataTypeStr=boolean
  AND{1,3..4,6,9..10} (6 alike) : Logic  Inputs=1  AllPortsSameDT=off  OutDataTypeStr=boolean
  AND8 : Logic  Inputs=4  AllPortsSameDT=off  OutDataTypeStr=boolean
  Abs{,1..2,4} (4 alike) : Abs
  Bus Creator : BusCreator  Inputs=15
  Bus Creator1 : BusCreator  Inputs=15
  Bus Selector : BusSelector  OutputSignals=PLAN_ALC_LcOverTkLe_ALCSwtOn,LeLineLcAvailable,PLAN_ALC_LcOverTkLe_LaneAvailable,PLAN_ALC_LcOverTkLe_PilotLaneAvailable,PLAN_ALC_LcOverTkLe_NoTurnLampReq,PLAN_ALC_LcOverTkLe_NoLcFinishFlag,PLAN_ALC_LcOverTkLe_dyDiff,PLAN_ALC_LcOverTkLe_IPVehSpd,PLAN_ALC_LcOverTkLe_LineValid,PLAN_ALC_LcOverTkLe_NotInDrvCancelArea,PLAN_ALC_LcOverTkLe_P0NotCutOut,PLAN_ALC_LcOverTkLe_OverTkTrigger,PLAN_ALC_LcOverTkLe_LineCurvatureValid  OutputAsBus=on
  Bus Selector1 : BusSelector  OutputSignals=PLAN_ALC_LcOverTkRi_ALCSwtOn,PLAN_ALC_LcOverTkRi_LaneAvailable,PLAN_ALC_LcOverTkRi_PilotLaneAvailable,PLAN_ALC_LcOverTkRi_NoTurnLampReq,PLAN_ALC_LcOverTkRi_NoLcFinishFlag,PLAN_ALC_LcOverTkRi_dyDiff,PLAN_ALC_LcOverTkRi_IPVehSpd,PLAN_ALC_LcOverTkRi_LineValid,PLAN_ALC_LcOverTkRi_NotInDrvCancelArea,PLAN_ALC_LcOverTkRi_P0NotCutOut,PLAN_ALC_LcOverTkRi_OverTkTrigger,PLAN_ALC_LcOverTkRi_LineCurvatureValid,RiLineLcAvailable  OutputAsBus=on
  Compare To Constant : simulink/Logic and Bit Operations/Compare To Constant  relop=>=  const=P_PLAN_ALC_vMinPreLC_OverTk  OutDataTypeStr=boolean
  Compare To Constant1 : simulink/Logic and Bit Operations/Compare To Constant  relop=>  const=0.1  OutDataTypeStr=boolean
  Compare To Constant10 : simulink/Logic and Bit Operations/Compare To Constant  relop===  const=6  OutDataTypeStr=boolean
  Compare To Constant11 : simulink/Logic and Bit Operations/Compare To Constant  relop=<  const=0.4  OutDataTypeStr=boolean
  Compare To Constant12 : simulink/Logic and Bit Operations/Compare To Constant  relop===  const=0  OutDataTypeStr=boolean
  Compare To Constant{2,5,7,13} (4 alike) : simulink/Logic and Bit Operations/Compare To Constant  relop=~=  const=0  OutDataTypeStr=boolean
  Compare To Constant14 : simulink/Logic and Bit Operations/Compare To Constant  relop===  const=0  OutDataTypeStr=boolean
  Compare To Constant15 : simulink/Logic and Bit Operations/Compare To Constant  relop=>=  const=P_PLAN_ALC_vMinPreLC_OverTk  OutDataTypeStr=boolean
  Compare To Constant16 : simulink/Logic and Bit Operations/Compare To Constant  relop=>  const=1  OutDataTypeStr=boolean
  Compare To Constant17 : simulink/Logic and Bit Operations/Compare To Constant  relop=<=  const=120  OutDataTypeStr=boolean
  Compare To Constant18 : simulink/Logic and Bit Operations/Compare To Constant  relop=>  const=1  OutDataTypeStr=boolean
  Compare To Constant19 : simulink/Logic and Bit Operations/Compare To Constant  relop=>  const=0  OutDataTypeStr=boolean
  Compare To Constant20 : simulink/Logic and Bit Operations/Compare To Constant  relop=<  const=0  OutDataTypeStr=boolean
  Compare To Constant21 : simulink/Logic and Bit Operations/Compare To Constant  relop=>  const=P_PLAN_ALC_DPCExtraMultiFrameConfirmCntOverTk  OutDataTypeStr=boolean
  Compare To Constant22 : simulink/Logic and Bit Operations/Compare To Constant  relop=>  const=P_PLAN_ALC_DPCExtraMultiFrameConfirmCntOverTk  OutDataTypeStr=boolean
  Compare To Constant3 : simulink/Logic and Bit Operations/Compare To Constant  relop=>  const=0.1  OutDataTypeStr=boolean
  Compare To Constant4 : simulink/Logic and Bit Operations/Compare To Constant  relop=<=  const=120  OutDataTypeStr=boolean
  Compare To Constant6 : simulink/Logic and Bit Operations/Compare To Constant  relop=<  const=0.4  OutDataTypeStr=boolean
  Compare To Constant8 : simulink/Logic and Bit Operations/Compare To Constant  relop===  const=7  OutDataTypeStr=boolean
  Compare To Constant9 : simulink/Logic and Bit Operations/Compare To Constant  relop=>=  const=P_PLAN_ALC_LcOverTkRearVehTTClimit  OutDataTypeStr=boolean
  Compare To Zero{,1..3} (4 alike) : simulink/Logic and Bit Operations/Compare To Zero  relop=~=  OutDataTypeStr=boolean
  Constant : Constant  Value=P_PLAN_ALC_PreCurvaturePreTime
  Constant1 : Constant  Value=P_PLAN_ALC_PreCurvatureFactor
  Counter1 : Subsystem
  Counter2 : Subsystem
  Divide : Product  Inputs=*/
  DocBlock : simulink/Model-Wide Utilities/DocBlock  DocumentType=Text
      content=|
      | 模块说明：
      | 该模块用于计算是否触发压速换道，换道条件如下：
      |
      | 当如下条件全部满足进入左换道状态
      | 1.自动超车换道开关开启；
      | 2.车身中心距离车道中心线0.4m以内；
      | 3.仪表车速大于等于60kmh；
      | 4.目标车道安全，换道过程中无碰撞风险；
      | 5.目标车道控制线有效持续5帧；
      | 6.存在P0；
      | 7.P0速度低于巡航设定车速DeltaSpd km/h；
      | 8.P0无向左侧切出倾向；
      | 9.左侧车道没有目标或目标车速高于P0 DeltaSpd km/h；
      | 10.车辆不在道路最左侧；
      | 11.距离跟车减速控制的剩余时间<=4s；
      | 13.距离上一次压速换道被驾驶员取消>1km；
      | 14.距离上一次换道时横向Override>1km；
      | 15.距离上一次换道(不区分意图)完成>5s；
      | 16.NOH未请求换道或巡航；
      | 17.转向灯未开启；
      | 18.上述条件均满足保持1.5s；
      |
      | 当如下条件全部满足进入右换道状态
      | 1.自动超车换道开关开启；
      | 2.车身中心距离车道中心线0.4m以内；
      | 3.仪表车速大于等于60kmh；
      | 4.右侧车道安全，换道过程中无碰撞风险；
      | 5.右侧车道控制线有效持续5帧；
      | 6.存在P0；
      | 7.P0速度低于巡航设定车速DeltaSpd km/h；
      | 8.P0无向左侧切出倾向；
      | 9.左侧车道没有目标或目标车速高于P0 DeltaSpd km/h；
      | 10.车辆在道路最左侧；
      | 11.距离跟车减速控制的剩余时间<=4s；
      | 13.距离上一次压速换道被驾驶员取消>1km；
      | 14.距离上一次换道时横向Override>1km；
      | 15.距离上一次换道(不区分意图)完成>5s；
      | 16.NOH未请求换道或巡航；
      | 17.转向灯未开启；
      | 18.上述条件均满足保持1.5s。
  DrvCancelSup : Subsystem
  Gain : Gain  Gain=1/3.6
  MATLAB Function : MATLAB Function  TreatAsAtomicUnit=on
  NOR : Logic  Operator=OR  AllPortsSameDT=off  OutDataTypeStr=boolean
  NOT{,1..3,6} (5 alike) : Logic  Operator=NOT  IconShape=distinctive  AllPortsSameDT=off  OutDataTypeStr=boolean
  NOT4 : Logic  Operator=NOR  AllPortsSameDT=off  OutDataTypeStr=boolean
  NOT5 : Logic  Operator=NOR  AllPortsSameDT=off  OutDataTypeStr=boolean
  OR : Logic  Operator=NOR  AllPortsSameDT=off  OutDataTypeStr=boolean
  OR1 : Logic  Operator=NOR  AllPortsSameDT=off  OutDataTypeStr=boolean
  OR2 : Logic  Operator=OR  AllPortsSameDT=off  OutDataTypeStr=boolean
  OR3 : Logic  Operator=OR  AllPortsSameDT=off  OutDataTypeStr=boolean
  Product : Product
  Product1 : Product
  Relational Operator2 : RelationalOperator  Operator=<=  OutDataTypeStr=boolean  RndMeth=Simplest
  Relational Operator3 : RelationalOperator  Operator=<=  OutDataTypeStr=boolean  RndMeth=Simplest
  Relational Operator4 : RelationalOperator  Operator=<=  OutDataTypeStr=boolean  RndMeth=Simplest
  Saturation : Saturate  UpperLimit=140  LowerLimit=10
  Subsystem : Subsystem
  Subsystem4 : Subsystem
  Subsystem5 : Subsystem
  Subtract : Sum  Inputs=+-
  TrueDurationTime2 : TrueDurationTime/TrueDurationTime  TCycle=0.02
  TrueDurationTime4 : TrueDurationTime/TrueDurationTime  TCycle=0.02
  TurnReqCal2 : MATLAB Function  Commented=on  TreatAsAtomicUnit=on
  LcOverTkLe : Outport
  LcOverTkRi : Outport  Port=2
  LcOverTkCancelLe : Outport  Port=3
  LcOverTkCancelRi : Outport  Port=4
  LcOverTkLeReady : Outport  Port=5
  LcOverTkRiReady : Outport  Port=6
  wires:
  LcAvRi/1 -> Bus Creator1/15
  LcAvLe/1 -> Bus Creator/15
  NOT6/1 -> [NoHighSpdObjAfter]
  AND8/1 -> NOT6/1
  Compare To Constant19/1 -> AND8/3
  Compare To Constant20/1 -> AND8/4
  Compare To Constant5/1 -> AND8/1
  Compare To Constant9/1 -> AND8/2
  Divide/1 -> Compare To Constant9/1
  Subtract/1 -> Abs2/1, Compare To Constant19/1
  Abs/1 -> Divide/1
  Abs2/1 -> Divide/2
  Dx/1 -> Abs/1, Compare To Constant20/1
  [Vego_kph] -> Subtract/2
  Vx/1 -> Subtract/1
  Valid/1 -> Compare To Constant5/1
  Compare To Constant21/1 -> Bus Creator/8  "PLAN_ALC_LcOverTkLe_DPC"
  [NoHighSpdObjAfter] -> Bus Creator1/9
  DPCRi/1 -> Relational Operator4/1
  [NoHighSpdObjAfter] -> Bus Creator/9
  DPCLe/1 -> Relational Operator3/1
  [DPCthreshold] -> Relational Operator3/2
  [Vego_kph] -> Compare To Constant17/1, Compare To Constant15/1
  Compare To Constant17/1 -> AND7/1
  Compare To Constant15/1 -> AND7/2
  Compare To Constant/1 -> AND/2
  Compare To Constant4/1 -> AND/1
  [DPCthreshold] -> Relational Operator4/2
  Subsystem/2(DPCthreshold) -> [DPCthreshold]
  [DeltaSpd] -> Subsystem5/10(DeltaSpd)
  Subsystem/1(DeltaSpd) -> [DeltaSpd]
  NOT2/1 -> [NoTurnLamp]
  Saturation/1 -> 1-D Lookup Table/1
  [LSM_PilotTurnSts] -> Compare To Constant8/1, Compare To Constant12/1
  [DrivingOnTheMostLeftLane_b] -> NOT/1
  DrivingOnTheMostLeftLane_b/1 -> [DrivingOnTheMostLeftLane_b]
  NOT/1 -> Bus Creator/2  "PLAN_ALC_LcOverTkLe_LaneAvailable"
  [LSM_PilotTurnSts] -> Compare To Constant14/1, Compare To Constant10/1
  LSM_PilotTurnSts/1 -> [LSM_PilotTurnSts]
  Compare To Constant14/1 -> OR3/1
  [DrivingOnTheMostLeftLane_b] -> Compare To Constant13/1
  Compare To Constant13/1 -> Bus Creator1/2  "PLAN_ALC_LcOverTkRi_LaneAvailable"
  Compare To Constant12/1 -> OR2/2
  Compare To Constant8/1 -> OR2/1
  Compare To Constant10/1 -> OR3/2
  [LineCurvatureValid] -> Compare To Zero3/1
  [LineCurvatureValid] -> Compare To Zero1/1
  Constant1/1 -> Product1/2
  MATLAB Function/1(curvature) -> Product1/1  "PLAN_ALC_PreCurvature"
  Compare To Zero3/1 -> Bus Creator/14  "PLAN_ALC_LcOverTkLe_LineCurvatureValid"
  Compare To Zero1/1 -> Bus Creator1/14  "PLAN_ALC_LcOverTkRi_LineCurvatureValid"
  Relational Operator2/1 -> [LineCurvatureValid]
  1-D Lookup Table/1 -> Relational Operator2/2
  [Vego_kph] -> Saturation/1
  Product1/1 -> Relational Operator2/1
  Constant/1 -> Product/2
  Product/1 -> MATLAB Function/3(x)
  Gain/1 -> Product/1
  [Vego_kph] -> Gain/1
  [HWALineC2] -> MATLAB Function/2(C2)
  [HWALineC1] -> MATLAB Function/1(C1)
  [LcOverTkSup_RiP0CutOut] -> NOT4/2
  [LcOverTkSup_LeP0CutOut] -> NOT5/2
  [LcOverTkSup_RiP0CutOut] -> NOT5/1
  LcCancelInCntRi/1 -> DrvCancelSup/3(CancelRi)
  Compare To Constant18/1 -> [LcFinishRi]
  Compare To Constant16/1 -> [LcFinishLe]
  ALC_sts/1 -> DrvCancelSup/8(ALC_sts)
  User_DrvOverride/1 -> DrvCancelSup/7(User_DrvOverride)
  Subsystem5/2(LcTriggerRi) -> [LcTriggerOverTkRi]
  Subsystem5/1(LcTriggerLe) -> [LcTriggerOverTkLe]
  User_ALC_Swt/1 -> Subsystem/1(User_ALC_Swt), [User_ALC_Swt]
  NearestObjSpeed_R/1 -> Subsystem5/9(NearestObjSpeed_R)
  NearestObjSpeed_L/1 -> Subsystem5/8(NearestObjSpeed_L)
  NearestObjValid_R/1 -> Subsystem5/7(NearestObjValid_R)
  NearestObjValid_L/1 -> Subsystem5/6(NearestObjValid_L)
  tStartDecel/1 -> Subsystem5/5(tStartDecel)
  P0Vr_ms/1 -> Subsystem5/3(P0Vr_ms)
  P0ID/1 -> Subsystem5/2(P0ID), [P0ID]
  SpdSetValue_kph/1 -> Subsystem5/1(SpdSetValue_kph)
  AND6/1 -> Bus Creator1/4  "PLAN_ALC_LcOverTkRi_NoTurnLampReq"
  OR3/1 -> Bus Creator1/3  "PLAN_ALC_LcOverTkRi_PilotLaneAvailable"
  [NoTurnLamp] -> AND1/1
  NOT5/1 -> Bus Creator1/12  "PLAN_ALC_LcOverTkRi_P0NotCutOut"
  NOT1/1 -> Bus Creator1/11  "PLAN_ALC_LcOverTkRi_NotInDrvCancelArea"
  [LcFinishLe] -> OR1/1
  [LcFinishRi] -> OR1/2
  [LcFinishRi] -> OR/2
  [LcFinishLe] -> OR/1
  [LcTriggerOverTkRi] -> Bus Creator1/13  "PLAN_ALC_LcOverTkRi_OverTkTrigger"
  [LcOveTkrSup_DrvCancel] -> NOT1/1
  [LcOverTkSup_LeP0CutOut] -> NOT4/1
  [LcOveTkrSup_DrvCancel] -> NOT3/1
  NOT4/1 -> Bus Creator/12  "PLAN_ALC_LcOverTkLe_P0NotCutOut"
  NOT3/1 -> Bus Creator/11  "PLAN_ALC_LcOverTkLe_NotInDrvCancelArea"
  LCKSts/1 -> DrvCancelSup/6(LCKsts)
  HWALineRange/1 -> Subsystem4/11(HWALineRange)
  HWALineC0/1 -> Subsystem4/10(HWALineC0)
  HWALineC1/1 -> Subsystem4/9(HWALineC1), [HWALineC1]
  HWALineC2/1 -> Subsystem4/8(HWALineC2), [HWALineC2]
  " HWALineC3"/1 -> Subsystem4/7(" HWALineC3")
  HWALineValid/1 -> Subsystem4/6(HWALineValid)
  LaneWidth/1 -> Subsystem4/5(LaneWidth)
  P0Vy/1 -> Subsystem4/4(P0Vy)
  P0Dy/1 -> Subsystem4/3(P0Dy)
  P0Dx/1 -> [P0Dx], Subsystem4/2(P0Dx)
  [Vego_kph] -> DrvCancelSup/5(V_ego)
  LcReason/1 -> DrvCancelSup/4(LcReason)
  LcCancelInCntLe/1 -> DrvCancelSup/2(CancelLe)
  [Vego_kph] -> Subsystem5/4(VehicleSpd_kph)  "VehicleSpd_kph"
  dyDiff/1 -> [dyDiff]
  LcFinishRi/1 -> Compare To Constant18/1
  Abs1/1 -> Compare To Constant6/1
  Vego_kph/1 -> [Vego_kph]
  Compare To Constant1/1 -> Bus Creator/10  "PLAN_ALC_LcOverTkLe_LineValid"
  [LcTriggerOverTkLe] -> Bus Creator/13  "PLAN_ALC_LcOverTkLe_OverTkTrigger"
  Bus Creator1/1 -> Bus Selector1/1, AND4/1  "LcfeRi"
  Compare To Constant3/1 -> Bus Creator1/10  "PLAN_ALC_LcOverTkRi_LineValid"
  Compare To Constant11/1 -> Bus Creator1/6  "PLAN_ALC_LcOverTkRi_dyDiff"
  LcFinishLe/1 -> Compare To Constant16/1
  [NoTurnLamp] -> AND6/1
  Compare To Constant6/1 -> Bus Creator/6  "PLAN_ALC_LcOverTkLe_dyDiff"
  Abs4/1 -> Compare To Constant11/1
  Compare To Zero2/1 -> TrueDurationTime4/1
  [dyDiff] -> Abs4/1
  OR1/1 -> Bus Creator1/5  "PLAN_ALC_LcOverTkRi_NoLcFinishFlag"
  Compare To Constant22/1 -> Bus Creator1/8  "PLAN_ALC_LcOverTkRi_DPC"
  HWALineLValid/1 -> Compare To Zero/1
  HWALineRValid/1 -> Compare To Zero2/1
  User_RightTurnLampReq/1 -> NOR/2
  Bus Creator/1 -> Bus Selector/1, AND3/1  "LcfeLe"
  TrueDurationTime2/1 -> Compare To Constant1/1
  AND1/1 -> Bus Creator/4  "PLAN_ALC_LcOverTkLe_NoTurnLampReq"
  TrueDurationTime4/1 -> Compare To Constant3/1
  OR/1 -> Bus Creator/5  "PLAN_ALC_LcOverTkLe_NoLcFinishFlag"
  [dyDiff] -> Abs1/1
  User_LeftTurnLampReq/1 -> NOR/1
  Compare To Zero/1 -> TrueDurationTime2/1
  AND/1 -> Bus Creator1/7  "PLAN_ALC_LcOverTkRi_IPVehSpd"
  AND7/1 -> Bus Creator/7  "PLAN_ALC_LcOverTkLe_IPVehSpd"
  [Vego_kph] -> Compare To Constant/1, Compare To Constant4/1
  NOR/1 -> DrvCancelSup/1(DrvTurnLamp), NOT2/1
  DrvCancelSup/1(OveTkrSup_DrvCancel) -> [LcOveTkrSup_DrvCancel]
  Subsystem4/1(LcOverTkSup_LeP0CutOut) -> [LcOverTkSup_LeP0CutOut]
  AND3/1 -> LcOverTkLe/1  "PLAN_ALC_LcOverTkLe"
  Subsystem4/2(LcOverTkSup_RiP0CutOut) -> [LcOverTkSup_RiP0CutOut]
  OR2/1 -> Bus Creator/3  "PLAN_ALC_LcOverTkLe_PilotLaneAvailable"
  AND4/1 -> LcOverTkRi/1  "PLAN_ALC_LcOverTkRi"
  [User_ALC_Swt] -> Compare To Constant2/1
  Compare To Constant2/1 -> Bus Creator/1  "PLAN_ALC_LcOverTkLe_ALCSwtOn"
  Compare To Constant7/1 -> Bus Creator1/1  "PLAN_ALC_LcOverTkRi_ALCSwtOn"
  [User_ALC_Swt] -> Compare To Constant7/1
  Subsystem5/3(LcOverTkCancelLe) -> LcOverTkCancelLe/1
  Subsystem5/4(LcOverTkCancelRi) -> LcOverTkCancelRi/1
  [P0ID] -> Subsystem4/1(P0ID)
  AND2/1 -> LcOverTkLeReady/1  "LcOverTkLeReady"
  Bus Selector/1 -> AND10/1
  Bus Selector1/1 -> AND9/1
  AND5/1 -> LcOverTkRiReady/1  "LcOverTkRiReady"
  Counter1/1(Cnt) -> Compare To Constant21/1
  Relational Operator3/1 -> Counter1/1(Trigger)
  Counter2/1(Cnt) -> Compare To Constant22/1
  Relational Operator4/1 -> Counter2/1(Trigger)
  [NoHighSpdObjAfter] -> AND2/2
  [NoHighSpdObjAfter] -> AND5/2
  AND9/1 -> AND5/1
  AND10/1 -> AND2/1
